simulink model "LCmodel"  (R2014a)
settings: Solver=FixedStepDiscrete  StartTime=0.0  StopTime=8000  RelTol=1e-3
undefined symbols (not defined in the file): material
libraries: identextras x30, simulink x16, slident x1
settings Model: Creator=md596  LastModifiedBy=md596

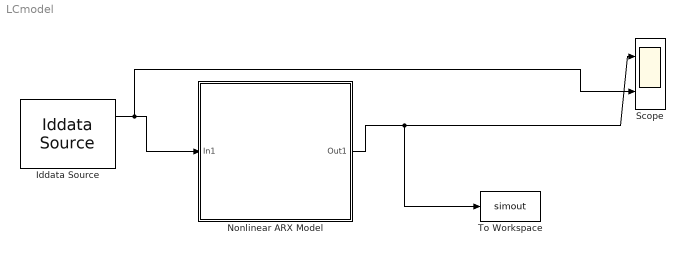
== system LCmodel ==
  Iddata Source : slident/Iddata Source  iddataobj=sine100Hz
  Nonlinear ARX Model : Subsystem  AncestorBlock=slident/Models/Nonlinear ARX Model  mask(Nonlinear ARX Model){sys=material, ICspec=Input and output values, X0=0, U0=0, Y0=0}
      mask prompts: sys "Model"; ICspec "Initial conditions:"; X0 "Specify initial states as a vector of 32 values."; U0 "Input level (scalar)"; Y0 "Output levels (scalar or vector of length equal to number of model outputs)"
      mask help:
      | Simulate a nonlinear ARX (idnlarx) model. Specify the name of an estimated idnlarx model for "Model". Specify initial conditions for simulation as one of the following:
      | 1. Steady-state (equilibrium) input and output signal levels.
      | 2. An initial state vector. Click on Help button for information on how to determine initial states from various requirements.
      mask init:
      | MaskVal = get_param(gcb,'MaskValues');
      | sysname = MaskVal{1};
      | if isa(sys,'idnlarx')
      |    maskEn = get_param(gcb,'MaskEnables');
      |    nu = size(sys,'nu');
      |    fInp = find_system(gcb,'FollowLinks','on','LookUnderMasks','all',...
      |       'SearchDepth',1,'Name','In1');
      |    
      |    if nu>0 && isempty(fInp)
      |       add_block('built-in/Inport',[gcb,'/In1'],'Position',[20   133    50   147])
      |    elseif nu==0 && ~isempty(fInp)
      |       delete_block(fInp);
      |    end
      |    %{
      |     if nu==0
      |         maskEn{4} = 'off';
      |     else
      |         maskEn{4} = 'on';
      |     end
      |    %}
      |    
      |    set_param(gcb,'MaskEnables',maskEn);
      |    
      | else
      |    sysname = '???';
      |    sys = [];
      |    U0 = [];
      |    Y0 = [];
      |    X0 = [];
      |    Nx = 0;   
      | end
      | 
      | if any(strcmp(get_param(bdroot(gcb),'SimulationStatus'),{'initializing','updating'}))
      |    lwarn = lastwarn;warn = warning('off');
      |    try
      |       [X0,Ts,WarnMsg] = idnlarxmaskinit('initialization',gcb,sys,ICspec,X0,U0,Y0);
      |       Nx = length(X0);
      |       warning(warn);lastwarn(lwarn);
      |       for i = 1:size(WarnMsg,1)
      |          warning(WarnMsg{i,1},WarnMsg{i,2})
      |       end
      |    catch E
      |       sys = [];
      |       U0 = [];
      |       Y0 = [];
      |       sysname = '???';
      |       X0 = [];
      |       Nx = 0;
      |       warning(warn);lastwarn(lwarn);
      |       throw(E)
      |    end
      | end
      mask Help: eval('identhelp(''idnlarx_block'')')
      mask Callback sys: idnlarxmaskinit('maskparamcallback',gcb)
      mask TypeOptions ICspec: Input and output values | State values
      mask Callback ICspec:
      | maskStr = get_param(gcb,'MaskValues');
      | if strcmp(maskStr{2}(1),'S')
      |     % "State values" option
      |     set_param(gcb,  'MaskVisibilities',   {'on';'on';'on';'off';'off'});
      |     %set_param(gcb,  'MaskEnables',        {'on';'on';'on';'off';'off'});
      | elseif strcmp(maskStr{2}(1),'I')
      |     % "Input and output values" option (default)
      |     set_param(gcb,  'MaskVisibilities',   {'on';'on';'off';'on';'on'});
      |     %set_param(gcb,  'MaskEnables',        {'on';'on';'off';'on';'on'});
      | end
      mask Display:
      | if strcmp(bdroot(gcb),'slident')
      |    disp('IDNLARX MODEL')
      | else
      |    disp(sysname)
      | end
  Scope : Scope  NumInputPorts=2
      settings: YMin=-5~-5  YMax=5~5
  To Workspace : ToWorkspace  VariableName=simout  SaveFormat=Timeseries  SampleTime=-1
  wires:
  Nonlinear ARX Model/1(Out1) -> Scope/1, To Workspace/1
  Iddata Source/1 -> Scope/2, Nonlinear ARX Model/1(In1)

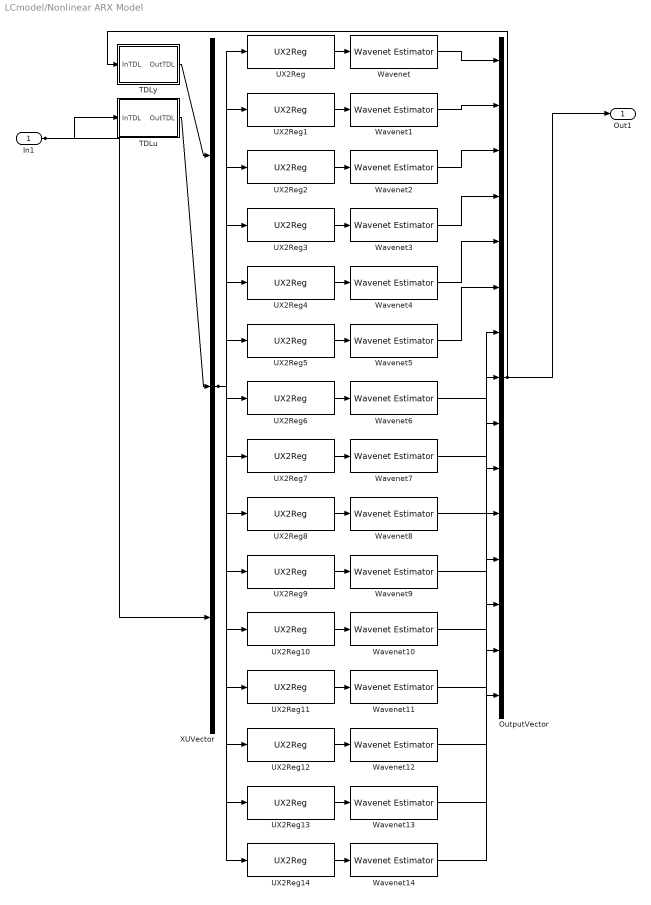
== system LCmodel/Nonlinear ARX Model ==
  In1 : Inport
  OutputVector : Concatenate  NumInputs=15
  TDLu : Subsystem
  TDLy : Subsystem
  UX2Reg : identextras/UX2Reg  ny=1  Nx=0  ynum=1  cumDel=0  ModelVar=[]  K=[1 0 0 0 0 0 0 0 0 0 0 0 0 0 0 0 0 0 0 0 0 0 0 0 0 0 0 0 0 0 0 0 0;0 1 0 0 0 0 0 0 0 0 0 0 0 0 0 0 0 0 0 0 0 0 0 0 0 0 0 0 0 0 0 0 0;0 0 0 0 0 0 0 0 0 0 0 0 0 0 0 0 0 0 0 0 0 0 0 0 0 0 0 0 0 0 1 0 0;0 0 0 0 0 0 0 0 0 0 0 0 0 0 0 0 0 0 0 0 0 0 0 0 0 0 0 0 0 0 0 1 0]
  UX2Reg1 : identextras/UX2Reg  ny=1  Nx=0  ynum=1  cumDel=0  ModelVar=[]  K=[0 0 1 0 0 0 0 0 0 0 0 0 0 0 0 0 0 0 0 0 0 0 0 0 0 0 0 0 0 0 0 0 0;0 0 0 1 0 0 0 0 0 0 0 0 0 0 0 0 0 0 0 0 0 0 0 0 0 0 0 0 0 0 0 0 0;0 0 0 0 0 0 0 0 0 0 0 0 0 0 0 0 0 0 0 0 0 0 0 0 0 0 0 0 0 0 1 0 0;0 0 0 0 0 0 0 0 0 0 0 0 0 0 0 0 0 0 0 0 0 0 0 0 0 0 0 0 0 0 0 1 0]
  UX2Reg10 : identextras/UX2Reg  ny=1  Nx=0  ynum=1  cumDel=0  ModelVar=[]  K=[0 0 0 0 0 0 0 0 0 0 0 0 0 0 0 0 0 0 0 0 1 0 0 0 0 0 0 0 0 0 0 0 0;0 0 0 0 0 0 0 0 0 0 0 0 0 0 0 0 0 0 0 0 0 1 0 0 0 0 0 0 0 0 0 0 0;0 0 0 0 0 0 0 0 0 0 0 0 0 0 0 0 0 0 0 0 0 0 0 0 0 0 0 0 0 0 1 0 0;0 0 0 0 0 0 0 0 0 0 0 0 0 0 0 0 0 0 0 0 0 0 0 0 0 0 0 0 0 0 0 1 0]
  UX2Reg11 : identextras/UX2Reg  ny=1  Nx=0  ynum=1  cumDel=0  ModelVar=[]  K=[0 0 0 0 0 0 0 0 0 0 0 0 0 0 0 0 0 0 0 0 0 0 1 0 0 0 0 0 0 0 0 0 0;0 0 0 0 0 0 0 0 0 0 0 0 0 0 0 0 0 0 0 0 0 0 0 1 0 0 0 0 0 0 0 0 0;0 0 0 0 0 0 0 0 0 0 0 0 0 0 0 0 0 0 0 0 0 0 0 0 0 0 0 0 0 0 1 0 0;0 0 0 0 0 0 0 0 0 0 0 0 0 0 0 0 0 0 0 0 0 0 0 0 0 0 0 0 0 0 0 1 0]
  UX2Reg12 : identextras/UX2Reg  ny=1  Nx=0  ynum=1  cumDel=0  ModelVar=[]  K=[0 0 0 0 0 0 0 0 0 0 0 0 0 0 0 0 0 0 0 0 0 0 0 0 1 0 0 0 0 0 0 0 0;0 0 0 0 0 0 0 0 0 0 0 0 0 0 0 0 0 0 0 0 0 0 0 0 0 1 0 0 0 0 0 0 0;0 0 0 0 0 0 0 0 0 0 0 0 0 0 0 0 0 0 0 0 0 0 0 0 0 0 0 0 0 0 1 0 0;0 0 0 0 0 0 0 0 0 0 0 0 0 0 0 0 0 0 0 0 0 0 0 0 0 0 0 0 0 0 0 1 0]
  UX2Reg13 : identextras/UX2Reg  ny=1  Nx=0  ynum=1  cumDel=0  ModelVar=[]  K=[0 0 0 0 0 0 0 0 0 0 0 0 0 0 0 0 0 0 0 0 0 0 0 0 0 0 1 0 0 0 0 0 0;0 0 0 0 0 0 0 0 0 0 0 0 0 0 0 0 0 0 0 0 0 0 0 0 0 0 0 1 0 0 0 0 0;0 0 0 0 0 0 0 0 0 0 0 0 0 0 0 0 0 0 0 0 0 0 0 0 0 0 0 0 0 0 1 0 0;0 0 0 0 0 0 0 0 0 0 0 0 0 0 0 0 0 0 0 0 0 0 0 0 0 0 0 0 0 0 0 1 0]
  UX2Reg14 : identextras/UX2Reg  ny=1  Nx=0  ynum=1  cumDel=0  ModelVar=[]  K=[0 0 0 0 0 0 0 0 0 0 0 0 0 0 0 0 0 0 0 0 0 0 0 0 0 0 0 0 1 0 0 0 0;0 0 0 0 0 0 0 0 0 0 0 0 0 0 0 0 0 0 0 0 0 0 0 0 0 0 0 0 0 1 0 0 0;0 0 0 0 0 0 0 0 0 0 0 0 0 0 0 0 0 0 0 0 0 0 0 0 0 0 0 0 0 0 1 0 0;0 0 0 0 0 0 0 0 0 0 0 0 0 0 0 0 0 0 0 0 0 0 0 0 0 0 0 0 0 0 0 1 0]
  UX2Reg2 : identextras/UX2Reg  ny=1  Nx=0  ynum=1  cumDel=0  ModelVar=[]  K=[0 0 0 0 1 0 0 0 0 0 0 0 0 0 0 0 0 0 0 0 0 0 0 0 0 0 0 0 0 0 0 0 0;0 0 0 0 0 1 0 0 0 0 0 0 0 0 0 0 0 0 0 0 0 0 0 0 0 0 0 0 0 0 0 0 0;0 0 0 0 0 0 0 0 0 0 0 0 0 0 0 0 0 0 0 0 0 0 0 0 0 0 0 0 0 0 1 0 0;0 0 0 0 0 0 0 0 0 0 0 0 0 0 0 0 0 0 0 0 0 0 0 0 0 0 0 0 0 0 0 1 0]
  UX2Reg3 : identextras/UX2Reg  ny=1  Nx=0  ynum=1  cumDel=0  ModelVar=[]  K=[0 0 0 0 0 0 1 0 0 0 0 0 0 0 0 0 0 0 0 0 0 0 0 0 0 0 0 0 0 0 0 0 0;0 0 0 0 0 0 0 1 0 0 0 0 0 0 0 0 0 0 0 0 0 0 0 0 0 0 0 0 0 0 0 0 0;0 0 0 0 0 0 0 0 0 0 0 0 0 0 0 0 0 0 0 0 0 0 0 0 0 0 0 0 0 0 1 0 0;0 0 0 0 0 0 0 0 0 0 0 0 0 0 0 0 0 0 0 0 0 0 0 0 0 0 0 0 0 0 0 1 0]
  UX2Reg4 : identextras/UX2Reg  ny=1  Nx=0  ynum=1  cumDel=0  ModelVar=[]  K=[0 0 0 0 0 0 0 0 1 0 0 0 0 0 0 0 0 0 0 0 0 0 0 0 0 0 0 0 0 0 0 0 0;0 0 0 0 0 0 0 0 0 1 0 0 0 0 0 0 0 0 0 0 0 0 0 0 0 0 0 0 0 0 0 0 0;0 0 0 0 0 0 0 0 0 0 0 0 0 0 0 0 0 0 0 0 0 0 0 0 0 0 0 0 0 0 1 0 0;0 0 0 0 0 0 0 0 0 0 0 0 0 0 0 0 0 0 0 0 0 0 0 0 0 0 0 0 0 0 0 1 0]
  UX2Reg5 : identextras/UX2Reg  ny=1  Nx=0  ynum=1  cumDel=0  ModelVar=[]  K=[0 0 0 0 0 0 0 0 0 0 1 0 0 0 0 0 0 0 0 0 0 0 0 0 0 0 0 0 0 0 0 0 0;0 0 0 0 0 0 0 0 0 0 0 1 0 0 0 0 0 0 0 0 0 0 0 0 0 0 0 0 0 0 0 0 0;0 0 0 0 0 0 0 0 0 0 0 0 0 0 0 0 0 0 0 0 0 0 0 0 0 0 0 0 0 0 1 0 0;0 0 0 0 0 0 0 0 0 0 0 0 0 0 0 0 0 0 0 0 0 0 0 0 0 0 0 0 0 0 0 1 0]
  UX2Reg6 : identextras/UX2Reg  ny=1  Nx=0  ynum=1  cumDel=0  ModelVar=[]  K=[0 0 0 0 0 0 0 0 0 0 0 0 1 0 0 0 0 0 0 0 0 0 0 0 0 0 0 0 0 0 0 0 0;0 0 0 0 0 0 0 0 0 0 0 0 0 1 0 0 0 0 0 0 0 0 0 0 0 0 0 0 0 0 0 0 0;0 0 0 0 0 0 0 0 0 0 0 0 0 0 0 0 0 0 0 0 0 0 0 0 0 0 0 0 0 0 1 0 0;0 0 0 0 0 0 0 0 0 0 0 0 0 0 0 0 0 0 0 0 0 0 0 0 0 0 0 0 0 0 0 1 0]
  UX2Reg7 : identextras/UX2Reg  ny=1  Nx=0  ynum=1  cumDel=0  ModelVar=[]  K=[0 0 0 0 0 0 0 0 0 0 0 0 0 0 1 0 0 0 0 0 0 0 0 0 0 0 0 0 0 0 0 0 0;0 0 0 0 0 0 0 0 0 0 0 0 0 0 0 1 0 0 0 0 0 0 0 0 0 0 0 0 0 0 0 0 0;0 0 0 0 0 0 0 0 0 0 0 0 0 0 0 0 0 0 0 0 0 0 0 0 0 0 0 0 0 0 1 0 0;0 0 0 0 0 0 0 0 0 0 0 0 0 0 0 0 0 0 0 0 0 0 0 0 0 0 0 0 0 0 0 1 0]
  UX2Reg8 : identextras/UX2Reg  ny=1  Nx=0  ynum=1  cumDel=0  ModelVar=[]  K=[0 0 0 0 0 0 0 0 0 0 0 0 0 0 0 0 1 0 0 0 0 0 0 0 0 0 0 0 0 0 0 0 0;0 0 0 0 0 0 0 0 0 0 0 0 0 0 0 0 0 1 0 0 0 0 0 0 0 0 0 0 0 0 0 0 0;0 0 0 0 0 0 0 0 0 0 0 0 0 0 0 0 0 0 0 0 0 0 0 0 0 0 0 0 0 0 1 0 0;0 0 0 0 0 0 0 0 0 0 0 0 0 0 0 0 0 0 0 0 0 0 0 0 0 0 0 0 0 0 0 1 0]
  UX2Reg9 : identextras/UX2Reg  ny=1  Nx=0  ynum=1  cumDel=0  ModelVar=[]  K=[0 0 0 0 0 0 0 0 0 0 0 0 0 0 0 0 0 0 1 0 0 0 0 0 0 0 0 0 0 0 0 0 0;0 0 0 0 0 0 0 0 0 0 0 0 0 0 0 0 0 0 0 1 0 0 0 0 0 0 0 0 0 0 0 0 0;0 0 0 0 0 0 0 0 0 0 0 0 0 0 0 0 0 0 0 0 0 0 0 0 0 0 0 0 0 0 1 0 0;0 0 0 0 0 0 0 0 0 0 0 0 0 0 0 0 0 0 0 0 0 0 0 0 0 0 0 0 0 0 0 1 0]
  Wavenet : identextras/Wavenet Estimator  Ts=1  NumReg=4  NumUnits=21  RegressorMean=[-0.026170808789716341 -0.026170575136221671 4.5253307596941399e-07 1.3575927959005618e-06]  NonLinearSubspace=[-0.10428579839314814 94.740310477045384 -3127.3391723294671 -1842.4431255477907;-0.10430423637203116 87.445766186952952 3499.154034800019 -964.72317536517983;-0.69128993933609262 10.420292877342458 -244.80792684004726 5689.719381753469;-0.69128715409179009 -37.906789183259775 188.62455205055861 -5266.2347018092751]  LinearSubspace=[-0.10428579839314814 94.740310477045384 -3127.3391723294671 -1842.4431255477907;-0.10430423637203116 87.445766186952952 3499.154034800019 -964.72317536517983;-0.69128993933609262 10.420292877342458 -244.80792684004726 5689.719381753469;-0.69128715409179009 -37.906789183259775 188.62455205055861 -5266.2347018092751]  OutputOffset=-0.026134092075233824  LinearCoef=[-0.10666271177114772;0.0055803336805429092;2.9737966329582914e-07;8.8200048380001776e-05]  ScalingCoef=[-3.2061896710205347e-05;0.00017585092676618036;-0.00014783083660797417;-0.00012830319803716007;-0.00012116011825072311;-0.0010198043083165605]  WaveletCoef=[2.6481133509969525e-05;-5.4645743309928117e-05;0.00011119627117632026;-7.2459861740940289e-05;2.9160529840565907e-05;6.7988059304699132e-05;3.1929359977342787e-05;-4.0167517159991064e-05;-4.4740838318038172e-05;-7.1958181174971555e-05;-4.4907645612946447e-05;-4.4667357816846083e-05;-4.4436342593452752e-05;-2.2489753462095122e-05;0.00023314946363089546]  ScalingDilation=[1;2;1;2;2;2]  WaveletDilation=[1;1;1;2;1;2;1;1;1;1;1;2;1;1;2]  ScalingTranslation=[1 1 0 2;-1 -1 0.5 0.5;1 -1 2 0;1.5 -0.5 -0.5 0.5;1 1 0.5 -0.5;-1 -1 0 0]  WaveletTranslation=[0 -1 1 -2;1 0 0 -1;0 1 0 0;-0.5 1.5 -0.5 -0.5;0 1 -1 -1;0.5 1.5 1 -1;-1 -1 0 0;-1 -1 -2 0;-1 1 0 -1;0 1 0 1;-1 -1 1 0;1 1 -0.5 -0.5;0 1 1 -1;0 -1 -1 -1;-1 -1 0 0]
  Wavenet1 : identextras/Wavenet Estimator  Ts=1  NumReg=4  NumUnits=18  RegressorMean=[-0.010580357246683464 -0.010580045708689277 4.5253307596941399e-07 1.3575927959005618e-06]  NonLinearSubspace=[-0.10369315575519288 97.160230479562742 -3146.572494883389 -1879.8313341325531;-0.10371108976937692 89.52238338734999 3538.4729848361712 -957.82408810961306;-0.69147236414052915 11.459642981278009 -262.65032307169372 5600.956018804407;-0.69146967090251688 -39.457032498680476 203.78996823219083 -5175.4166915086844]  LinearSubspace=[-0.10369315575519288 97.160230479562742 -3146.572494883389 -1879.8313341325531;-0.10371108976937692 89.52238338734999 3538.4729848361712 -957.82408810961306;-0.69147236414052915 11.459642981278009 -262.65032307169372 5600.956018804407;-0.69146967090251688 -39.457032498680476 203.78996823219083 -5175.4166915086844]  OutputOffset=-0.010551340155272568  LinearCoef=[-0.10602339606056921;0.0054211332184346522;-6.4989499113362857e-06;8.8949538743363646e-05]  ScalingCoef=-0.00010891652905379222  WaveletCoef=[5.2074998969280323e-06;5.69611247123473e-05;-8.7964667642088194e-05;-9.1060221199863641e-05;7.9918776859858353e-06;-3.2682746664049887e-05;5.2547236162162488e-05;-4.1162918861847826e-05;3.6893538258882873e-05;-5.0341850029336054e-05;3.9688407818650693e-05;-1.7684732092945445e-05;-4.3843456393274247e-05;-3.835297498222734e-05;3.0106692889838803e-05;-2.2695003470780008e-05;-3.0283300770763568e-05]  ScalingDilation=1  WaveletDilation=[1;1;1;2;1;1;2;2;1;1;2;1;1;1;2;1;2]  ScalingTranslation=[1 1 0 2]  WaveletTranslation=[-1 -1 0 0;0 1 0 0;1 0 0 -1;-0.5 -1.5 0.5 0.5;-1 -1 0 1;-1 1 0 -1;1.5 0 0 -0.5;-0.5 1.5 -0.5 0;0 1 -1 -1;1 -1 2 0;0 -1.5 0 0.5;0 -1 -1 0;-1 -1 1 0;-1 -1 -1 0;0.5 1.5 1 -1;1 -1 -1 1;0 -1.5 0.5 0]
  Wavenet10 : identextras/Wavenet Estimator  Ts=1  NumReg=4  NumUnits=2  RegressorMean=[-0.0070114963302030514 -0.0070114963302030497 4.5253307596941399e-07 1.3575927959005618e-06]  NonLinearSubspace=[-0.013716300559618878 -146.8407534142207 971.40310669039616 4486.6651840899458;-0.013718538432040316 -134.60293046645668 4371.3123998399924 -1402.0557736517553;-0.70675696237711672 -309.19207069551044 -1224.120167528456 -783.74964548148648;-0.70675691413513753 314.65460275104948 1120.4182954819983 723.88994902165564]  LinearSubspace=[-0.013716300559618878 -146.8407534142207 971.40310669039616 4486.6651840899458;-0.013718538432040316 -134.60293046645668 4371.3123998399924 -1402.0557736517553;-0.70675696237711672 -309.19207069551044 -1224.120167528456 -783.74964548148648;-0.70675691413513753 314.65460275104948 1120.4182954819983 723.88994902165564]  OutputOffset=-0.0070110279648434477  LinearCoef=[-0.013723723954726512;-0.00067237684615929273;-4.8757684769940774e-06;-2.3653210944023022e-06]  ScalingCoef=zeros(0,1)  WaveletCoef=[2.5167426689596489e-05;-1.644974671881232e-05]  ScalingDilation=zeros(0,1)  WaveletDilation=[2;1]  ScalingTranslation=zeros(0,4)  WaveletTranslation=[-1.5 0.5 0 0;-1 0 1 -1]
  Wavenet11 : identextras/Wavenet Estimator  Ts=1  NumReg=4  NumUnits=5  RegressorMean=[-0.0018828019995777456 -0.0018827630573284254 4.5253307596941399e-07 1.3575927959005618e-06]  NonLinearSubspace=[-0.030389316993387195 -190.30024464690069 -3214.3199147172018 3015.1358127306821;-0.030395420741272276 -177.32009609515669 3550.9092761621646 2611.2659911920364;-0.70571443524547794 -142.0443094529025 -67.533987238219865 -3584.4990725809512;-0.70571416767976813 157.87628775668125 53.00915968592755 3342.1949001509042]  LinearSubspace=[-0.030389316993387195 -190.30024464690069 -3214.3199147172018 3015.1358127306821;-0.030395420741272276 -177.32009609515669 3550.9092761621646 2611.2659911920364;-0.70571443524547794 -142.0443094529025 -67.533987238219865 -3584.4990725809512;-0.70571416767976813 157.87628775668125 53.00915968592755 3342.1949001509042]  OutputOffset=-0.0018794887245718167  LinearCoef=[-0.030447963695254102;-0.001789901565542688;-4.298553949541528e-06;-5.7481505344835382e-05]  ScalingCoef=-0.00012104953114210255  WaveletCoef=[3.0628557356388261e-05;-2.5576542181758999e-05;2.7144772567891699e-05;-1.5607038597781084e-05]  ScalingDilation=1  WaveletDilation=[1;1;1;1]  ScalingTranslation=[1 -1 0 2]  WaveletTranslation=[0 -1 0 1;1 -1 -2 1;1 0 0 -2;-1 0 0 1]
  Wavenet12 : identextras/Wavenet Estimator  Ts=1  NumReg=4  NumUnits=6  RegressorMean=[-0.0098288510466421532 -0.009828812104392912 4.5253307596941399e-07 1.3575927959005618e-06]  NonLinearSubspace=[-0.039417234233220112 177.97955372149465 -3212.2750759715623 2806.2812967363075;-0.039424846420925655 165.37601601076437 3574.0658518924201 2328.8747911541286;-0.70481855378832081 102.645640915051 -97.176169894870625 -4096.2838646571536;-0.70481812340979544 -121.84978666217005 76.904335330844162 3809.075564392901]  LinearSubspace=[-0.039417234233220112 177.97955372149465 -3212.2750759715623 2806.2812967363075;-0.039424846420925655 165.37601601076437 3574.0658518924201 2328.8747911541286;-0.70481855378832081 102.645640915051 -97.176169894870625 -4096.2838646571536;-0.70481812340979544 -121.84978666217005 76.904335330844162 3809.075564392901]  OutputOffset=-0.0098212798905174641  LinearCoef=[-0.039550139371055858;0.0022398688945682306;-6.0958362220835603e-06;-6.8610133337735285e-05]  ScalingCoef=9.4526271649301993e-05  WaveletCoef=[-3.0898609577241692e-05;-3.9615976709700103e-05;2.6211542434851841e-05;-2.4619928028306274e-05;-2.2940629735304532e-05]  ScalingDilation=2  WaveletDilation=[1;1;2;2;1]  ScalingTranslation=[-1 -1 -0.5 0]  WaveletTranslation=[0 -1 -1 0;-1 -1 2 0;1.5 0 0 0.5;-1.5 0 0 -0.5;-1 0 -1 1]
  Wavenet13 : identextras/Wavenet Estimator  Ts=1  NumReg=4  NumUnits=14  RegressorMean=[-0.0032022820785459084 -0.0032022431362965917 4.5253307596941399e-07 1.3575927959005618e-06]  NonLinearSubspace=[-0.045050927786639355 166.04819926118233 -3260.6143296402443 -2683.825589875215;-0.045059746765122255 154.44353173226568 3623.5522047803361 -2169.7917536616569;-0.70414055477320658 80.154417775274524 -113.69054758236975 4490.8434006751222;-0.7041399859316787 -100.66150123459465 90.424464575714538 -4180.2850605932344]  LinearSubspace=[-0.045050927786639355 166.04819926118233 -3260.6143296402443 -2683.825589875215;-0.045059746765122255 154.44353173226568 3623.5522047803361 -2169.7917536616569;-0.70414055477320658 80.154417775274524 -113.69054758236975 4490.8434006751222;-0.7041399859316787 -100.66150123459465 90.424464575714538 -4180.2850605932344]  OutputOffset=-0.003191076737913395  LinearCoef=[-0.045243114391565538;0.0025717853634977328;1.5671094705960978e-06;7.6504925400941475e-05]  ScalingCoef=-9.9822396179775273e-05  WaveletCoef=[3.5276937550264067e-05;-4.8328706595462109e-05;-3.7141422988927842e-05;-2.5326390085233877e-05;-3.0692147766751746e-05;3.0048063943822975e-05;-2.8204061052384078e-05;-3.1647151066128787e-05;-2.0423050845983386e-05;-2.6470617729436721e-05;-3.1720106960421532e-05;2.158505231072561e-05;-2.3698132530195086e-05]  ScalingDilation=2  WaveletDilation=[1;2;1;1;1;1;2;1;2;1;1;1;1]  ScalingTranslation=[-1.5 0 1 0]  WaveletTranslation=[0 1 0 0;1 1 -0.5 -0.5;0 -1 0 0;1 -1 -2 0;1 -1 2 0;0 1 -1 -1;-0.5 1.5 -0.5 -0.5;-1 -1 -2 0;-1.5 0 0 0.5;-1 -1 2 0;-1 0 0 -1;-1 -1 0 -1;0 1 0 2]
  Wavenet14 : identextras/Wavenet Estimator  Ts=1  NumReg=4  NumUnits=11  RegressorMean=[-0.0072768095792888517 -0.0072767316947903041 4.5253307596941399e-07 1.3575927959005618e-06]  NonLinearSubspace=[-0.048136817702923149 167.27372814356156 -3153.1626420611224 2584.2342427936451;-0.04814554091210297 154.69286027885278 3573.1583692456966 1963.8875721756879;-0.70373022699786603 80.674743980694089 -154.08768610894788 -4188.287467735121;-0.70372962571786324 -102.70002802895301 125.31479695726937 3877.1641104611958]  LinearSubspace=[-0.048136817702923149 167.27372814356156 -3153.1626420611224 2584.2342427936451;-0.04814554091210297 154.69286027885278 3573.1583692456966 1963.8875721756879;-0.70373022699786603 80.674743980694089 -154.08768610894788 -4188.287467735121;-0.70372962571786324 -102.70002802895301 125.31479695726937 3877.1641104611958]  OutputOffset=-0.0072737398433942984  LinearCoef=[-0.048363441737585451;0.0025674250695098019;-1.1098595737625341e-05;-7.2694828038644168e-05]  ScalingCoef=-0.00011523343841972339  WaveletCoef=[-1.8188481531684392e-05;-2.5815291033268017e-05;-2.594801606719508e-05;-2.2821814432964493e-05;4.9211885011069102e-05;4.1741994757568959e-05;5.3869405428018938e-05;-2.4576674679173511e-05;2.9162057732762418e-05;-1.9384614084612905e-05]  ScalingDilation=2  WaveletDilation=[1;2;1;2;1;1;2;1;2;1]  ScalingTranslation=[-1.5 0 0 -0.5]  WaveletTranslation=[0 1 0 0;-0.5 -1.5 0 -0.5;0 -1 -1 0;1 1 0.5 0;0 1 1 0;0 1 -1 0;0.5 1.5 0 0.5;0 -1 1 0;-1 -1 0.5 0;1 1 0 1]
  Wavenet2 : identextras/Wavenet Estimator  Ts=1  NumReg=4  NumUnits=31  RegressorMean=[-0.010922231488911034 -0.010922036777664729 4.5253307596941399e-07 1.3575927959005618e-06]  NonLinearSubspace=[-0.095731880508939604 106.82582965108249 -3163.0125822293048 -1981.7576820717145;-0.095748046750634364 98.233472955962327 3600.995032921775 -984.40809558748822;-0.69381328359970318 16.962514682107319 -298.70228947969224 5254.2713675142113;-0.69381104899944468 -45.258891128176046 238.18663356575868 -4844.9945172981124]  LinearSubspace=[-0.095731880508939604 106.82582965108249 -3163.0125822293048 -1981.7576820717145;-0.095748046750634364 98.233472955962327 3600.995032921775 -984.40809558748822;-0.69381328359970318 16.962514682107319 -298.70228947969224 5254.2713675142113;-0.69381104899944468 -45.258891128176046 238.18663356575868 -4844.9945172981124]  OutputOffset=-0.010920295085140024  LinearCoef=[-0.097544791820450533;0.0048806525211832867;-1.1833805531388439e-05;7.2926308973288929e-05]  ScalingCoef=[0.00011233161687753791;-0.00013965738271145534;0.00087718105393504219;0.0001665010016854602]  WaveletCoef=[-2.2583874310435015e-05;-3.9018578646723749e-05;2.6550826747408826e-05;-7.566286202699e-05;5.3444807612638866e-05;-0.00014044984584376266;-6.5211726056507325e-05;-0.00011316794829290204;8.2949324704050331e-05;-8.7238709220014077e-05;-5.1819386183583586e-05;-6.4851681527748115e-05;8.1662815006723708e-06;-7.680538643080731e-05;2.2040924971326318e-05;-7.1935488944660647e-05;1.999501773154729e-05;6.3910891341308491e-05;3.5007300398756379e-05;5.3524410063664412e-05;2.4601619462997696e-05;-4.5799706640354331e-05;1.9106686546178533e-05;-2.6877019604335747e-05;6.9344059596979633e-05;-5.3811725012248463e-05;-2.9533716503162065e-05]  ScalingDilation=[2;2;2;2]  WaveletDilation=[1;1;1;1;2;2;1;1;2;2;2;2;1;2;1;1;2;1;1;1;1;2;1;2;1;2;2]  ScalingTranslation=[-1 1 0 -0.5;1.5 -0.5 -0.5 0.5;0.5 1.5 -0.5 -0.5;-1 1 0 -1]  WaveletTranslation=[0 1 0 0;-1 -1 1 0;1 0 0 0;0 -1 -1 0;0.5 1.5 0.5 -0.5;0.5 1.5 -0.5 -0.5;1 -1 1 0;1 1 0 -1;0.5 -1.5 0.5 0;0 -1.5 0.5 0;-0.5 1.5 0.5 -0.5;-0.5 1.5 -0.5 -0.5;0 1 -1 -1;-0.5 -1.5 -0.5 0.5;0 -1 -1 1;-1 1 0 -1;0 -1.5 -0.5 0;0 1 0 -1;-1 1 -1 0;0 1 1 0;-1 1 0 1;1 -1 0 1;0 -1 0 0;-0.5 -1.5 0.5 0.5;0 -1 0 1;-0.5 -1.5 0.5 1;1 -1 0 0]
  Wavenet3 : identextras/Wavenet Estimator  Ts=1  NumReg=4  NumUnits=7  RegressorMean=[0.00023678667173222278 0.00023698138297908734 4.5253307596941399e-07 1.3575927959005618e-06]  NonLinearSubspace=[-0.088468248025774743 124.6190836799572 -3084.3818056868972 -2218.2065412140432;-0.088481728747536251 113.5729071034511 3711.8268587383432 -810.63668572262316;-0.69577364439350997 28.245331409507894 -482.42060146627813 4506.1440064623557;-0.69577192615733119 -58.534003462833631 402.56947255494197 -4121.0183221599127]  LinearSubspace=[-0.088468248025774743 124.6190836799572 -3084.3818056868972 -2218.2065412140432;-0.088481728747536251 113.5729071034511 3711.8268587383432 -810.63668572262316;-0.69577364439350997 28.245331409507894 -482.42060146627813 4506.1440064623557;-0.69577192615733119 -58.534003462833631 402.56947255494197 -4121.0183221599127]  OutputOffset=0.00021089870388248591  LinearCoef=[-0.089906049028649071;0.004132814807450336;-1.4453334438197808e-05;8.9956980598168696e-05]  ScalingCoef=0.00044180690730852328  WaveletCoef=[7.4147170552966234e-05;1.3137447428159116e-05;4.3302416021154673e-05;4.2539415576271475e-05;-2.6663155069069766e-05;-9.0359729777685771e-05]  ScalingDilation=1  WaveletDilation=[1;1;1;1;1;1]  ScalingTranslation=[0 2 1 -1]  WaveletTranslation=[1 -1 0 -3;0 1 0 0;0 1 -2 -1;0 -1 1 -2;0 1 0 2;0 1 1 -1]
  Wavenet4 : identextras/Wavenet Estimator  Ts=1  NumReg=4  NumUnits=17  RegressorMean=[-0.016098552318771015 -0.016098357607525041 4.5253307596941399e-07 1.3575927959005618e-06]  NonLinearSubspace=[-0.086761796532893218 129.8862723673854 -3010.7819579121165 -2223.1390610830372;-0.086774598380439438 118.01525143212005 3637.4664987709421 -881.05416939252143;-0.69621023790499859 32.12022551640964 -453.48456143525669 4384.3521340249508;-0.69620863834838198 -63.01605555162898 375.32104184615599 -3997.5002153214887]  LinearSubspace=[-0.086761796532893218 129.8862723673854 -3010.7819579121165 -2223.1390610830372;-0.086774598380439438 118.01525143212005 3637.4664987709421 -881.05416939252143;-0.69621023790499859 32.12022551640964 -453.48456143525669 4384.3521340249508;-0.69620863834838198 -63.01605555162898 375.32104184615599 -3997.5002153214887]  OutputOffset=-0.016106548128003245  LinearCoef=[-0.088122517935663378;0.0039181403789806035;-1.9187818183436176e-06;7.5550316778759494e-05]  ScalingCoef=zeros(0,1)  WaveletCoef=[5.9331587752804419e-05;3.8291915355884714e-05;5.2562890487862508e-05;5.5479368103724201e-05;-9.3351897760792174e-05;7.7276581775900834e-05;4.874012206210669e-05;-3.0902298453329491e-05;-3.5760265596179547e-05;2.3485415640938249e-05;-2.7021885551801038e-05;-3.671505480487062e-05;-3.0447366258703963e-05;-5.1630355886089396e-05;-3.9690390544313416e-05;-2.8308169237767772e-05;2.4158186262562443e-05]  ScalingDilation=zeros(0,1)  WaveletDilation=[1;1;2;2;1;1;1;1;2;2;1;2;1;2;2;2;1]  ScalingTranslation=zeros(0,4)  WaveletTranslation=[0 1 0 0;0 -1 0 -2;0.5 1.5 -0.5 -1;0.5 1.5 0.5 -1;0 1 0 -1;0 1 -1 -1;0 1 1 -1;-1 -1 1 0;-0.5 1.5 -0.5 -0.5;1.5 0 0 0.5;-1 -1 -1 -1;1 -1 -1 0.5;1 -1 0 -1;-0.5 -1.5 -0.5 0;0 -1.5 0.5 0.5;1 -1 0 0.5;0 -1 0 0]
  Wavenet5 : identextras/Wavenet Estimator  Ts=1  NumReg=4  NumUnits=12  RegressorMean=[-0.0042931706924166542 -0.0042930149234193804 4.5253307596941399e-07 1.3575927959005618e-06]  NonLinearSubspace=[-0.079778153759883882 135.51225622343225 -3035.7364393715911 -2241.912052350468;-0.079790281156589038 123.46928739441299 3616.6616859440419 -1078.6153123372578;-0.69790303897968475 37.790366452255235 -376.91674642610087 4397.5308237127183;-0.69790164841198887 -67.397144664950829 310.44823999347091 -4017.9465241223352]  LinearSubspace=[-0.079778153759883882 135.51225622343225 -3035.7364393715911 -2241.912052350468;-0.079790281156589038 123.46928739441299 3616.6616859440419 -1078.6153123372578;-0.69790303897968475 37.790366452255235 -376.91674642610087 4397.5308237127183;-0.69790164841198887 -67.397144664950829 310.44823999347091 -4017.9465241223352]  OutputOffset=-0.0042844780407264652  LinearCoef=[-0.080841175623241029;0.0037022108909321684;-7.1385005319176025e-07;6.997624816627435e-05]  ScalingCoef=[0.00027210284993585675;0.00014913309299885625]  WaveletCoef=[3.540604118081127e-05;4.9040661947897942e-05;-3.9716031647802736e-05;-2.9801852876145567e-05;3.0846602299828612e-05;-3.5747366626221375e-05;4.2522394636773249e-05;3.1837273300367729e-05;-4.7612894561981298e-05;3.9597233568851245e-05]  ScalingDilation=[2;2]  WaveletDilation=[1;2;1;1;2;1;2;2;1;2]  ScalingTranslation=[0 1.5 -0.5 -0.5;-1 1 0 0]  WaveletTranslation=[0 -1 0 -2;0.5 1.5 0.5 -0.5;-1 -1 1 0;-1 -1 -1 0;-1 -1 0 0.5;1 -1 0 -1;0.5 -1.5 0 -0.5;1.5 0 -1 -0.5;-1 1 0 -1;-1 1 0 -1]
  Wavenet6 : identextras/Wavenet Estimator  Ts=1  NumReg=4  NumUnits=10  RegressorMean=[-0.0081407039368402261 -0.0081405092255938671 4.5253307596941399e-07 1.3575927959005618e-06]  NonLinearSubspace=[-0.076465000327932672 -145.02220460041312 2896.6341096030692 -2360.4121798532183;-0.076476054253887066 -131.51706771319633 -3628.7097345447078 -893.84890472822838;-0.69865384140383624 -46.459387543157355 513.95776868016549 3954.9335745028279;-0.69865262721563537 76.727771164346947 -433.77822284243007 -3598.7592130074104]  LinearSubspace=[-0.076465000327932672 -145.02220460041312 2896.6341096030692 -2360.4121798532183;-0.076476054253887066 -131.51706771319633 -3628.7097345447078 -893.84890472822838;-0.69865384140383624 -46.459387543157355 513.95776868016549 3954.9335745028279;-0.69865262721563537 76.727771164346947 -433.77822284243007 -3598.7592130074104]  OutputOffset=-0.0081509400541381147  LinearCoef=[-0.077392964285158697;-0.003409201245144529;4.4574471133986349e-06;6.9723509506734827e-05]  ScalingCoef=0.00050949344454248276  WaveletCoef=[5.0723697799964928e-05;5.1843270043013739e-05;-2.8578740266127856e-05;-7.9686702658023843e-05;2.5783378261662363e-05;4.2218316242917685e-05;3.334094918547977e-05;-2.3657007422736766e-05;-0.00010100172220609476]  ScalingDilation=2  WaveletDilation=[1;2;1;2;1;2;2;2;2]  ScalingTranslation=[-0.5 1.5 0.5 1]  WaveletTranslation=[0 1 0 -2;0.5 -1.5 -0.5 -0.5;-1 0 0 -1;-0.5 1.5 0.5 0.5;-1 -1 1 0;0.5 -1.5 0.5 -1;1.5 0 0 -0.5;-1.5 0 0 0.5;-0.5 1.5 0.5 1]
  Wavenet7 : identextras/Wavenet Estimator  Ts=1  NumReg=4  NumUnits=16  RegressorMean=[-0.0067215312982888235 -0.0067213755292916469 4.5253307596941399e-07 1.3575927959005618e-06]  NonLinearSubspace=[-0.086974480309407812 123.02750025646402 -3069.1391674852262 -2123.5042767967216;-0.086988181573670373 112.45925243076358 3610.6131097852931 -947.67571263098523;-0.69615628209736258 27.528814921870477 -382.51481439248209 4612.6232090286385;-0.69615456612251236 -56.951772127335907 314.79532994841537 -4228.9162483533664]  LinearSubspace=[-0.086974480309407812 123.02750025646402 -3069.1391674852262 -2123.5042767967216;-0.086988181573670373 112.45925243076358 3610.6131097852931 -947.67571263098523;-0.69615628209736258 27.528814921870477 -382.51481439248209 4612.6232090286385;-0.69615456612251236 -56.951772127335907 314.79532994841537 -4228.9162483533664]  OutputOffset=-0.0067171327299120733  LinearCoef=[-0.088338934429115654;0.0041557124431391753;-1.8486543119377897e-05;7.7604934471511467e-05]  ScalingCoef=-0.00010678465071949776  WaveletCoef=[3.2588246173907357e-05;1.8050294808289876e-05;5.693009167293732e-05;4.6836525826071531e-05;-4.7227118830317108e-05;4.2345657650199593e-05;4.9032653727043839e-05;3.0878784531503995e-05;-3.3175672317531759e-05;-3.760059051224308e-05;-3.580978304738033e-05;-3.7401744550528663e-05;-3.8598338966086772e-05;2.3251518459755072e-05;-2.6492826691417006e-05]  ScalingDilation=2  WaveletDilation=[1;1;2;2;1;1;2;2;1;1;1;2;2;1;2]  ScalingTranslation=[1.5 -0.5 -0.5 0.5]  WaveletTranslation=[0 1 0 0;0 -1 0 -2;0.5 1.5 -0.5 -1;0.5 1.5 0.5 -0.5;-1 -1 0 0;0 1 2 0;1.5 0 0 0;-1 -1 0 0;1 0 0 -1;0 -1 -2 0;0 -1 2 1;-0.5 -1.5 -0.5 0.5;-0.5 -1.5 0.5 0.5;-1 -1 0 1;1 -1 0 0.5]
  Wavenet8 : identextras/Wavenet Estimator  Ts=1  NumReg=4  NumUnits=17  RegressorMean=[-0.025157493690587347 -0.025157376863840123 4.5253307596941399e-07 1.3575927959005618e-06]  NonLinearSubspace=[-0.052898749075599313 185.7995223427771 -2802.2984292594106 2912.9550393023637;-0.05290575089030651 166.96831313491953 3794.1001807115781 1396.6395500405904;-0.70304269198051128 111.38564997106836 -493.85928521233558 -3285.5778244598118;-0.70304216051768775 -137.93058075538656 419.19608853754198 2961.3011189487024]  LinearSubspace=[-0.052898749075599313 185.7995223427771 -2802.2984292594106 2912.9550393023637;-0.05290575089030651 166.96831313491953 3794.1001807115781 1396.6395500405904;-0.70304269198051128 111.38564997106836 -493.85928521233558 -3285.5778244598118;-0.70304216051768775 -137.93058075538656 419.19608853754198 2961.3011189487024]  OutputOffset=-0.025158497053816061  LinearCoef=[-0.053184995925954055;0.0021489380410069461;-9.4055614838254128e-06;-4.3713424495866335e-05]  ScalingCoef=[-5.0965859672832233e-05;0.00020767450000677492]  WaveletCoef=[-3.1266534897908534e-05;-6.0569177372577952e-05;4.7304830991615844e-05;-2.7613660483090076e-05;-3.9562221810889451e-05;-2.7136356033362659e-05;-2.5705315472732822e-05;2.9290659077969517e-05;-5.1614347177085404e-05;3.1374527342806319e-05;-2.9448968897639264e-05;5.1620429379578995e-05;2.5685541721108478e-05;4.2085668817676698e-05;3.5898306761497376e-05]  ScalingDilation=[2;2]  WaveletDilation=[1;2;2;1;1;1;1;1;1;1;2;2;1;1;1]  ScalingTranslation=[1 1 -0.5 0;1.5 0 0 0.5]  WaveletTranslation=[0 1 0 0;-0.5 -1.5 0 -0.5;0.5 -1.5 0 -0.5;-1 0 0 1;0 -1 -1 0;1 -1 1 0;1 1 -1 -2;0 -1 0 1;1 0 0 1;-1 -1 0 -1;-1.5 0 0 -0.5;0.5 1.5 0 0.5;-1 1 0 0;0 1 1 0;0 1 -1 0]
  Wavenet9 : identextras/Wavenet Estimator  Ts=1  NumReg=4  NumUnits=19  RegressorMean=[-0.0026035059520311907 -0.0026035059520311903 4.5253307596941399e-07 1.3575927959005618e-06]  NonLinearSubspace=[-0.052518225474227138 195.2183449114232 -1911.8510004246418 3544.5075794584513;-0.052524204526205452 172.40524917703826 4011.4968068068983 367.89550788166656;-0.70310010596160388 138.12242552285275 -1133.8240612694819 -2646.5388113856779;-0.70309965474680913 -165.58372751106751 976.95704465141228 2354.2993377795065]  LinearSubspace=[-0.052518225474227138 195.2183449114232 -1911.8510004246418 3544.5075794584513;-0.052524204526205452 172.40524917703826 4011.4968068068983 367.89550788166656;-0.70310010596160388 138.12242552285275 -1133.8240612694819 -2646.5388113856779;-0.70309965474680913 -165.58372751106751 976.95704465141228 2354.2993377795065]  OutputOffset=-0.0026258228554534636  LinearCoef=[-0.052801486641741752;0.0018537667403401412;-9.5312366585506977e-06;-3.4018704423864805e-05]  ScalingCoef=[-0.0001182382656385628;0.00038654336665662253;-0.00050544246673519524]  WaveletCoef=[8.4809746001939808e-05;2.2894748294303133e-05;-3.8828558622972656e-05;-0.00012008288918680129;5.7336553686644278e-05;-4.4921449268668192e-05;-3.3247165987431355e-05;4.1254524845821116e-05;2.988789598151967e-05;-3.6880920124581168e-05;-3.9271945006019079e-05;-2.0040998287282355e-05;4.2054013481360133e-05;4.0051189551320922e-05;-2.6995573026181489e-05;2.6263335078551781e-05]  ScalingDilation=[2;1;2]  WaveletDilation=[1;1;2;1;2;1;1;2;1;2;2;1;2;1;2;2]  ScalingTranslation=[1.5 -0.5 -0.5 -0.5;0 1 -1 -1;-0.5 1.5 0 0.5]  WaveletTranslation=[0 1 0 0;0 -1 1 2;-1.5 0 0 0;0 1 -1 -1;-0.5 1.5 0 0.5;1 1 0 0;1 -1 1 0;1.5 0 0 0;0 1 -1 1;-0.5 -1.5 0 -0.5;-0.5 -1.5 -1 0;1 -1 -1 1;-1 1 0 1;0 2 1 1;-1.5 0 -0.5 -1;1.5 0 1 -0.5]
  XUVector : Concatenate  NumInputs=3
  Out1 : Outport
  wires:
  TDLy/1(OutTDL) -> XUVector/1
  TDLu/1(OutTDL) -> XUVector/2
  In1/1 -> XUVector/3, TDLu/1(InTDL)
  XUVector/1 -> UX2Reg/1, UX2Reg1/1, UX2Reg2/1, UX2Reg3/1, UX2Reg4/1, UX2Reg5/1, UX2Reg6/1, UX2Reg7/1, UX2Reg8/1, UX2Reg9/1, UX2Reg10/1, UX2Reg11/1, UX2Reg12/1, UX2Reg13/1, UX2Reg14/1
  UX2Reg/1 -> Wavenet/1
  Wavenet/1 -> OutputVector/1
  UX2Reg1/1 -> Wavenet1/1
  Wavenet1/1 -> OutputVector/2
  UX2Reg2/1 -> Wavenet2/1
  Wavenet2/1 -> OutputVector/3
  UX2Reg3/1 -> Wavenet3/1
  Wavenet3/1 -> OutputVector/4
  UX2Reg4/1 -> Wavenet4/1
  Wavenet4/1 -> OutputVector/5
  UX2Reg5/1 -> Wavenet5/1
  Wavenet5/1 -> OutputVector/6
  UX2Reg6/1 -> Wavenet6/1
  Wavenet6/1 -> OutputVector/7
  UX2Reg7/1 -> Wavenet7/1
  Wavenet7/1 -> OutputVector/8
  UX2Reg8/1 -> Wavenet8/1
  Wavenet8/1 -> OutputVector/9
  UX2Reg9/1 -> Wavenet9/1
  Wavenet9/1 -> OutputVector/10
  UX2Reg10/1 -> Wavenet10/1
  Wavenet10/1 -> OutputVector/11
  UX2Reg11/1 -> Wavenet11/1
  Wavenet11/1 -> OutputVector/12
  UX2Reg12/1 -> Wavenet12/1
  Wavenet12/1 -> OutputVector/13
  UX2Reg13/1 -> Wavenet13/1
  Wavenet13/1 -> OutputVector/14
  UX2Reg14/1 -> Wavenet14/1
  Wavenet14/1 -> OutputVector/15
  OutputVector/1 -> Out1/1, TDLy/1(InTDL)

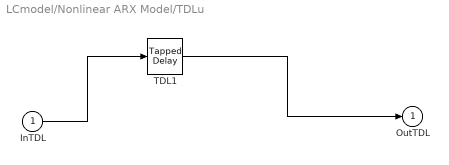
== system LCmodel/Nonlinear ARX Model/TDLu ==
  InTDL : Inport
  TDL1 : simulink/Discrete/Tapped Delay  vinit=[0;0]  samptime=1  NumDelays=2  DelayOrder=Newest  includeCurrent=off
  OutTDL : Outport
  wires:
  InTDL/1 -> TDL1/1
  TDL1/1 -> OutTDL/1

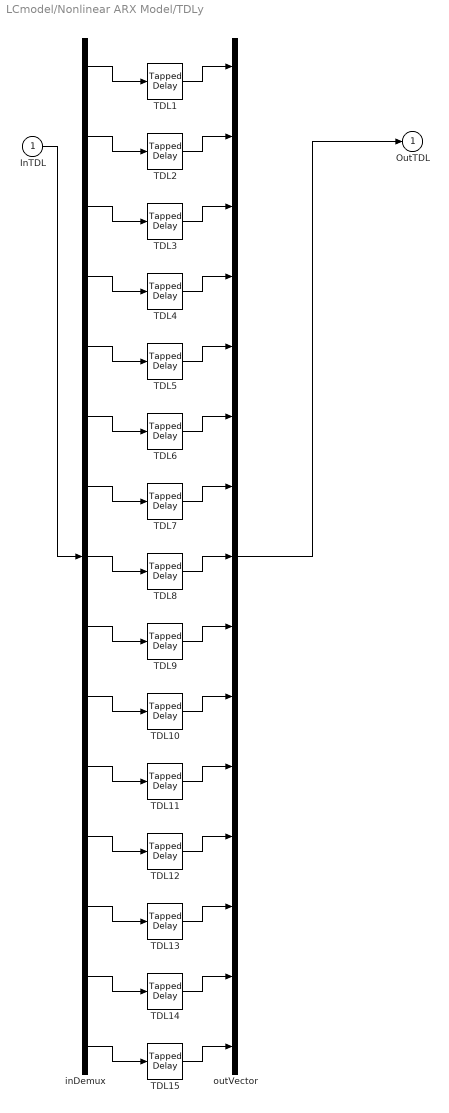
== system LCmodel/Nonlinear ARX Model/TDLy ==
  InTDL : Inport
  TDL{1..15} (15 alike) : simulink/Discrete/Tapped Delay  vinit=[0;0]  samptime=1  NumDelays=2  DelayOrder=Newest  includeCurrent=off
  inDemux : Demux  Outputs=15
  outVector : Concatenate  NumInputs=15
  OutTDL : Outport
  wires:
  InTDL/1 -> inDemux/1
  outVector/1 -> OutTDL/1
  inDemux/1 -> TDL1/1
  TDL1/1 -> outVector/1
  inDemux/2 -> TDL2/1
  TDL2/1 -> outVector/2
  inDemux/3 -> TDL3/1
  TDL3/1 -> outVector/3
  inDemux/4 -> TDL4/1
  TDL4/1 -> outVector/4
  inDemux/5 -> TDL5/1
  TDL5/1 -> outVector/5
  inDemux/6 -> TDL6/1
  TDL6/1 -> outVector/6
  inDemux/7 -> TDL7/1
  TDL7/1 -> outVector/7
  inDemux/8 -> TDL8/1
  TDL8/1 -> outVector/8
  inDemux/9 -> TDL9/1
  TDL9/1 -> outVector/9
  inDemux/10 -> TDL10/1
  TDL10/1 -> outVector/10
  inDemux/11 -> TDL11/1
  TDL11/1 -> outVector/11
  inDemux/12 -> TDL12/1
  TDL12/1 -> outVector/12
  inDemux/13 -> TDL13/1
  TDL13/1 -> outVector/13
  inDemux/14 -> TDL14/1
  TDL14/1 -> outVector/14
  inDemux/15 -> TDL15/1
  TDL15/1 -> outVector/15
